simulink model "Exemplu2_pag4"  (R2021b)
settings: Solver=VariableStepAuto  StartTime=0.0  StopTime=5000  RelTol=1e-10
undefined symbols (not defined in the file): kR
settings Model: Creator=alexandra.szedlak-st  LastModifiedBy=alexandra.szedlak-st

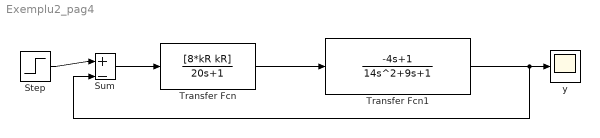
== system Exemplu2_pag4 ==
  Step : Step  Time=0  After=5  SampleTime=0
  Sum : Sum  Inputs=|+-
  Transfer Fcn : TransferFcn  Numerator=[8*kR kR]  Denominator=[20 1]
  Transfer Fcn1 : TransferFcn  Numerator=[-4 1]  Denominator=[14 9 1]
  y : Scope
  wires:
  Transfer Fcn/1 -> Transfer Fcn1/1
  Sum/1 -> Transfer Fcn/1
  Transfer Fcn1/1 -> Sum/2, y/1
  Step/1 -> Sum/1
